simulink library "INT_FlFltCtl_Ht"  (R2016b)
settings: Solver=VariableStepAuto  StartTime=0.0  StopTime=10.0  RelTol=1e-3
settings Model: Creator=liutao  LastModifiedBy=liutao

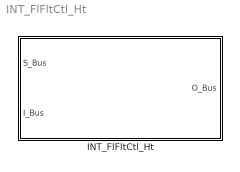
== system INT_FlFltCtl_Ht ==
  INT_FlFltCtl_Ht : Subsystem

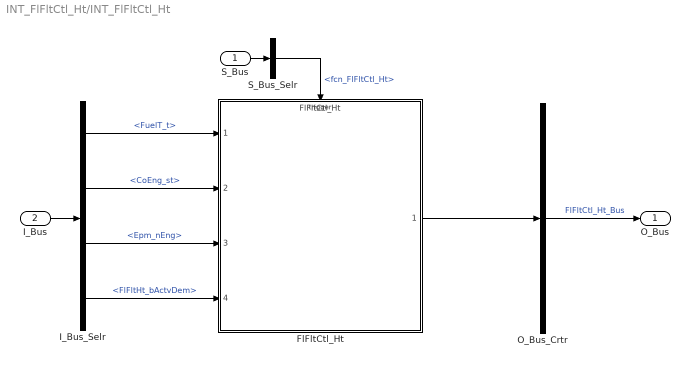
== system INT_FlFltCtl_Ht/INT_FlFltCtl_Ht ==
  S_Bus : Inport
  I_Bus : Inport  Port=2
  FlFltCtl_Ht : ModelReference  ModelNameDialog=FlFltCtl_Ht  SimulationMode=Normal  ModelReferenceVersion=1.8  TriggerPortName=function  TriggerPortTriggerType=function-call  TriggerPortStatesWhenEnabling=held
  I_Bus_Selr : BusSelector  OutputSignals=FuelT_t,CoEng_st,Epm_nEng,FlFltHt_bActvDem
  O_Bus_Crtr : BusCreator  Inputs=1
  S_Bus_Selr : BusSelector  OutputSignals=fcn_FlFltCtl_Ht
  O_Bus : Outport
  wires:
  S_Bus_Selr/1 -> FlFltCtl_Ht/Trigger  "<fcn_FlFltCtl_Ht>"
  S_Bus/1 -> S_Bus_Selr/1
  I_Bus/1 -> I_Bus_Selr/1
  I_Bus_Selr/1 -> FlFltCtl_Ht/1  "<FuelT_t>"
  I_Bus_Selr/2 -> FlFltCtl_Ht/2  "<CoEng_st>"
  I_Bus_Selr/3 -> FlFltCtl_Ht/3  "<Epm_nEng>"
  I_Bus_Selr/4 -> FlFltCtl_Ht/4  "<FlFltHt_bActvDem>"
  O_Bus_Crtr/1 -> O_Bus/1  "FlFltCtl_Ht_Bus"
  FlFltCtl_Ht/1 -> O_Bus_Crtr/1
